simulink model "practica_PDCAN_GRAV"  (R2017b)
settings: Solver=VariableStepAuto  StartTime=0.0  StopTime=20  RelTol=1e-3
settings Model: Creator=god_z  LastModifiedBy=god_z

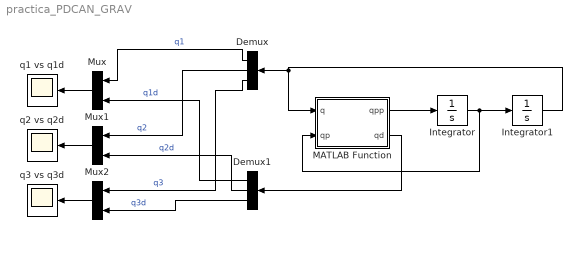
== system practica_PDCAN_GRAV ==
  Demux : Demux  Outputs=3
  Demux1 : Demux  Outputs=3
  Integrator : Integrator
  Integrator1 : Integrator
  MATLAB Function : MATLAB Function  TreatAsAtomicUnit=on
  Mux : Mux  Inputs=2
  Mux1 : Mux  Inputs=2
  Mux2 : Mux  Inputs=2
  q1 vs q1d : Scope
  q2 vs q2d : Scope
  q3 vs q3d : Scope
  wires:
  MATLAB Function/1(qpp) -> Integrator/1
  Integrator/1 -> Integrator1/1, MATLAB Function/2(qp)
  Integrator1/1 -> MATLAB Function/1(q), Demux/1
  MATLAB Function/2(qd) -> Demux1/1
  Mux2/1 -> q3 vs q3d/1
  Mux1/1 -> q2 vs q2d/1
  Mux/1 -> q1 vs q1d/1
  Demux/1 -> Mux/1  "q1"
  Demux/2 -> Mux1/1  "q2"
  Demux/3 -> Mux2/1  "q3"
  Demux1/1 -> Mux/2  "q1d"
  Demux1/2 -> Mux1/2  "q2d"
  Demux1/3 -> Mux2/2  "q3d"

== matlab function practica_PDCAN_GRAV/MATLAB Function ==
  data: q input; qpp output; qp input; qd output
function [qpp, qd] = fcn(q, qp)
    %#codegen
    % Asume que q y qp son vectores columna de tamaño 3
    assert(isvector(q) && numel(q) == 3, 'q debe ser un vector de tamaño 3');
    assert(isvector(qp) && numel(qp) == 3, 'qp debe ser un vector de tamaño 3');

    %% Parámetros del sistema 
    I1 = 0.1;
    I3 = 0.1;
    l3 = 1;
    l1 = 1;
    m2 = 0.2;
    m3 = 0.2;

    q1 = q(1);
    q2 = q(2);
    q3 = q(3);

    q1p = qp(1);
    q2p = qp(2);
    q3p = qp(3);

    M = [I1 + m3 * (l3 * l3) * cos(q3) * cos(q3), 0, 0;
         0, m2 + m3, 1/2 * m3 * l3 * cos(q3);
         0, 1/2 * m3 * l3 * cos(q3), m3 * (l3 * l3) + I3];

    C = [-m3 * (l3 * l3) * sin(2 * q3) * q3p, 0, 0;
         0, 0, -1/2 * m3 * l3 * sin(q3) * q3p;
         1/2 * m3 * (l3 * l3) * sin(2 * q3) * q1p, 0, 0];

    g = [0; m2 + m3; m3 * l3 * cos(q3)];

    %% Control 
    p = 2;
    d = 1;

    qd = [1; 0.5; 0.5];
    qtilde = q - qd;
    tau = -p * qtilde - d * qp + g;

    %% Modelo dinámico 
    qpp = pinv(M) * (tau - C * qp - g);

    % Especificar tamaños de salida
    qpp = reshape(qpp, [3, 1]); % Tamaño esperado: columna de tamaño 3
    qd = reshape(qd, [3, 1]);   % Tamaño esperado: columna de tamaño 3
end
